simulink model "RC_Circuit_R2020a"  (R2020b)
settings: Solver=VariableStepAuto  StartTime=0.0  StopTime=10.0  MaxStep=1e-3  RelTol=1e-3
values from neighbouring files (symbols this model uses):
  RC = 1*10^3*1*10^-6    (= 0.001)    [RC_Circuit.m]
libraries: simulink x1
settings Model: Creator=hp  LastModifiedBy=hp
settings DebuggingCC: UnconnectedInputMsg=none  UnconnectedOutputMsg=none  UnconnectedLineMsg=none
settings ModelReferenceCC: EnableRefExpFcnMdlSchedulingChecks=off

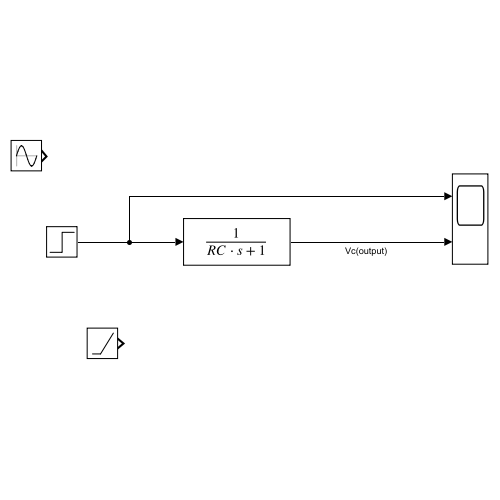
[thumbnail: Simulink's stored preview of the top-level diagram]
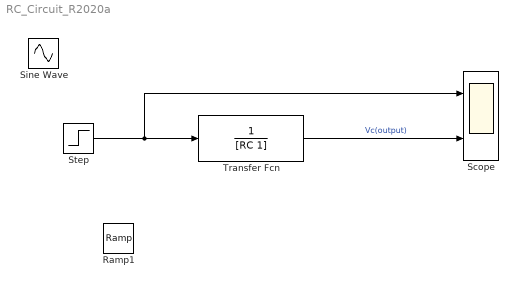
== system RC_Circuit_R2020a ==
  Ramp1 : simulink/Sources/Ramp  slope=1  start=1  InitialOutput=0
  Scope : Scope  NumInputPorts=2
  Sine Wave : Sin  Amplitude=5  Frequency=2*pi  SampleTime=0
  Step : Step  SampleTime=0
  Transfer Fcn : TransferFcn  Denominator=[RC 1]
  wires:
  Transfer Fcn/1 -> Scope/2  "Vc(output)"
  Step/1 -> Scope/1, Transfer Fcn/1
